simulink model "controlador"  (R2018a)
settings: Solver=VariableStepAuto  StartTime=0.0  StopTime=10.0  RelTol=1e-3
values from neighbouring files (symbols this model uses):
  K1 = [21.6 3 -5; 2.9 19 -4]*10e-4    [codigo_ex.m]    (also in controlador.m = [0.0216    0.0030   -0.0050; prueba_controlador_cpp.m = [0.0216    0.0030   -0.0050; sistema_tanques_control.m; tank_mod.m)
  K2 = [-0.95 -0.32; -0.3 -0.91]*10e-4    [codigo_ex.m]    (also in controlador.m = 1.0e-03 *K2; prueba_controlador_cpp.m = 1.0e-03 *K2; sistema_tanques_control.m; tank_mod.m)
  q_max = 1.5*10e-4    (= 0.0015)    [codigo_ex.m]    (also in controlador.m; prueba_controlador_cpp.m; sistema_tanques_control.m; tank_mod.m)
  q_min = 0    [codigo_ex.m]    (also in controlador.m; prueba_controlador_cpp.m; sistema_tanques_control.m; tank_mod.m)
  tm = 1    [codigo_ex.m]    (also in sistema_tanques_control.m; tank_mod.m)
libraries: instrumentlib x1
settings Model: Creator=carma  LastModifiedBy=carma

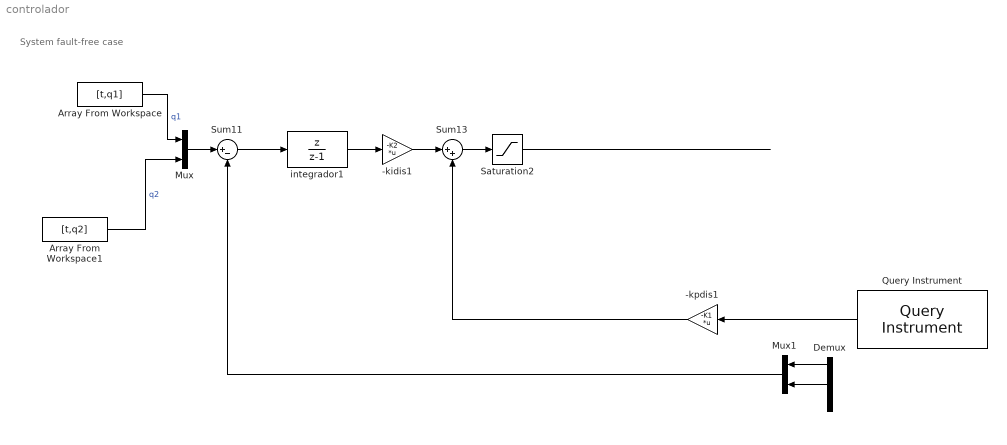
== system controlador ==
  note: System fault-free case
  -kidis1 : Gain  Gain=-K2  Multiplication=Matrix(K*u) (u vector)  SampleTime=tm
  -kpdis1 : Gain  Gain=-K1  Multiplication=Matrix(K*u) (u vector)  SampleTime=tm
  Array From Workspace : FromWorkspace  VariableName=[t,q1]  SampleTime=0
  Array From Workspace1 : FromWorkspace  VariableName=[t,q2]  SampleTime=0
  Demux : Demux  Outputs=3
  Mux : Mux  Inputs=2
  Mux1 : Mux  Inputs=2
  Query Instrument : instrumentlib/Query Instrument  sampleTime=1  isWorkspaceObject=off  timeout=10  inputBufferSize=512  protocol=Serial  serialPort=COM1  baudRate=115200  gpibVendor=Keysight Technologies  boardIndex=0  primaryAddress=1  secondaryAddress=0  visaVendor=Keysight  visaSerialPort=0  chassisIndex=0  logicalAddress=0  tcpRemoteHost='127.0.0.1'  tcpRemotePort=4500  udpRemoteHost='127.0.0.1'  udpRemotePort=9090  visaTCPBoardIndex=0  visaTCPRemoteHost='127.0.0.1'  usbBoardIndex=0  usbManufID=0  usbModelCode=0  usbSerialNumber=0  initAction=None  initCommand='DATA:SOURCE CH1'  initFunction=get  queryCommand=''  responseFormat=ASCII  asciiFormatting='%f,%f\n'  precision=8-bit integer  byteOrder=Little endian  valuesToRead=1  removeBytes=on  afterOutputAction=Repeat query for new data  enableFrames=on  frameSize=2
      settings: SourceProductName=Instrument Control Toolbox  SourceProductBaseCode=IC
  Saturation2 : Saturate  UpperLimit=q_max  LowerLimit=q_min
  Sum11 : Sum  Inputs=|+-  SampleTime=tm
  Sum13 : Sum  Inputs=|++  SampleTime=tm
  integrador1 : DiscreteTransferFcn  Numerator=[1 0]  Denominator=[1 -1]  SampleTime=tm
  wires:
  Demux/2 -> Mux1/2
  Array From Workspace/1 -> Mux/1  "q1"
  integrador1/1 -> -kidis1/1
  Mux/1 -> Sum11/1
  Saturation2/1 -> ?
  Mux1/1 -> Sum11/2
  Array From Workspace1/1 -> Mux/2  "q2"
  Demux/1 -> Mux1/1
  Sum11/1 -> integrador1/1
  Sum13/1 -> Saturation2/1
  -kidis1/1 -> Sum13/1
  -kpdis1/1 -> Sum13/2
  Query Instrument/1 -> -kpdis1/1
